simulink model "average_inverter_foc"  (R2023b)
settings: Solver=FixedStepAuto  StartTime=0.0  StopTime=simcfg.stop_time  FixedStep=simcfg.Ts_plant  RelTol=1e-3
InitFcn:
  | motor_control_params
values from neighbouring files (symbols this model uses):
  control = evalin('base', 'control')    [build_vibration_comp_test.m]    (also in evaluate_vibration_comp_test.m; motor_control_params.m = apply_cogging_load_config(control, cogging_load_config); open_cogging_position_scan_model.m = apply_cogging_load_config(control, cfg); open_position_scan_ff_validation_model.m = apply_cogging_load_config(control, cfg))
undefined symbols (not defined in the file or in its folder): inverter, motor, simcfg
libraries: mcbplantlib x1, autolibpmsmexterior x1
settings Model: Creator=user  LastModifiedBy=user

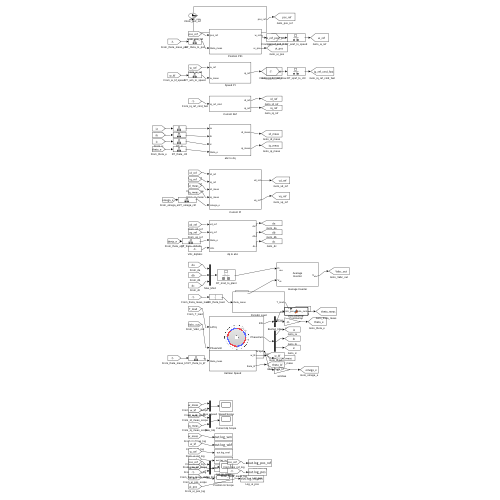
[thumbnail: Simulink's stored preview of the top-level diagram]
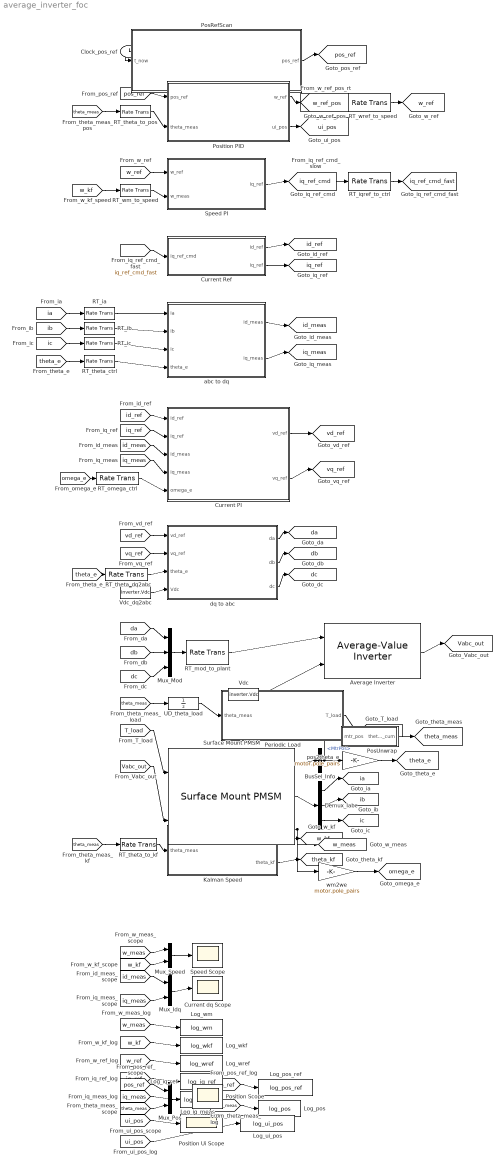
== system average_inverter_foc ==
  Average Inverter : mcbplantlib/Average-Value Inverter
  BusSel_Info : BusSelector  OutputSignals=MtrPos
  Clock_pos_ref : Clock
  Current PI : Subsystem
  Current Ref : Subsystem
  Current dq Scope : Scope
  Demux_Iabc : Demux  Outputs=3
  Kalman Speed : Subsystem
  Log_iq_meas : ToWorkspace  VariableName=log_iq_meas  SaveFormat=Timeseries  SampleTime=-1
  Log_iq_ref : ToWorkspace  VariableName=log_iq_ref  SaveFormat=Timeseries  SampleTime=-1
  Log_pos : ToWorkspace  VariableName=log_pos  SaveFormat=Timeseries  SampleTime=-1
  Log_pos_ref : ToWorkspace  VariableName=log_pos_ref  SaveFormat=Timeseries  SampleTime=-1
  Log_ui_pos : ToWorkspace  VariableName=log_ui_pos  SaveFormat=Timeseries  SampleTime=-1
  Log_wkf : ToWorkspace  VariableName=log_wkf  SaveFormat=Timeseries  SampleTime=-1
  Log_wm : ToWorkspace  VariableName=log_wm  SaveFormat=Timeseries  SampleTime=-1
  Log_wref : ToWorkspace  VariableName=log_wref  SaveFormat=Timeseries  SampleTime=-1
  Mux_Idq : Mux  Inputs=2
  Mux_Mod : Mux  Inputs=3
  Mux_Pos : Mux  Inputs=2
  Mux_Speed : Mux  Inputs=2
  Periodic Load : Subsystem
  PosRefScan : Subsystem
  PosUnwrap : MATLAB Function  TreatAsAtomicUnit=on
  Position PID : Subsystem
  Position Scope : Scope
  Position Ui Scope : Scope
  RT_ia : RateTransition  OutPortSampleTime=simcfg.Ts_ctrl
  RT_ib : RateTransition  OutPortSampleTime=simcfg.Ts_ctrl
  RT_ic : RateTransition  OutPortSampleTime=simcfg.Ts_ctrl
  RT_iqref_to_ctrl : RateTransition  OutPortSampleTime=simcfg.Ts_ctrl
  RT_mod_to_plant : RateTransition  OutPortSampleTime=simcfg.Ts_plant
  RT_omega_ctrl : RateTransition  OutPortSampleTime=simcfg.Ts_ctrl
  RT_theta_ctrl : RateTransition  OutPortSampleTime=simcfg.Ts_ctrl
  RT_theta_dq2abc : RateTransition  OutPortSampleTime=simcfg.Ts_ctrl
  RT_theta_to_kf : RateTransition  OutPortSampleTime=simcfg.Ts_ctrl
  RT_theta_to_pos : RateTransition  OutPortSampleTime=simcfg.Ts_pos
  RT_wm_to_speed : RateTransition  OutPortSampleTime=simcfg.Ts_speed
  RT_wref_to_speed : RateTransition  OutPortSampleTime=simcfg.Ts_speed
  Speed PI : Subsystem
  Speed Scope : Scope
  Surface Mount PMSM : autolibpmsmexterior/Surface Mount PMSM  port_config=Torque  sim_type=Discrete  Ts=simcfg.Ts_plant  P=motor.pole_pairs  Rs=motor.Rs  Ldq_=motor.Ld  KConstText=Permanent flux linkage constant (lambda_pm):  lambda_pm=motor.psi_f  Ke=159.9771  Kt=1.323  mechanical=[motor.J, motor.B, 0]  idq0=[0 0]  theta_init=0  omega_init=0  KConst=motor.psi_f  lambda_pm_calc=motor.psi_f  RefBlkName='autolibpmsmexterior/Surface Mount PMSM'  aMode=5  Ldq="[0.0017      0.0017]"
  UD_theta_load : UnitDelay  SampleTime=simcfg.Ts_plant  HasFrameUpgradeWarning=on
  Vdc : Constant  Value=inverter.Vdc
  Vdc_dq2abc : Constant  Value=inverter.Vdc
  abc to dq : Subsystem
  dq to abc : Subsystem
  pos2theta_e : Gain  Gain=motor.pole_pairs
  wm2we : Gain  Gain=motor.pole_pairs
  tag scope: T_load=global, Vabc_out=global, da=global, db=global, dc=global, ia=global, ib=global, ic=global, id_meas=global, id_ref=global, iq_meas=global, iq_ref=global, iq_ref_cmd=global, iq_ref_cmd_fast=global, omega_e=global, pos_ref=global, theta_e=global, theta_kf=global, theta_meas=global, ui_pos=global, vd_ref=global, vq_ref=global, w_kf=global, w_meas=global, w_ref=global, w_ref_pos=global
  wires:
  Clock_pos_ref/1 -> PosRefScan/1(t_now)
  PosRefScan/1(pos_ref) -> [pos_ref]
  [theta_meas] -> RT_theta_to_pos/1
  [pos_ref] -> Position PID/1(pos_ref)
  RT_theta_to_pos/1 -> Position PID/2(theta_meas)
  Position PID/1(w_ref) -> [w_ref_pos]
  Position PID/2(ui_pos) -> [ui_pos]
  [w_ref_pos] -> RT_wref_to_speed/1
  RT_wref_to_speed/1 -> [w_ref]
  [w_kf] -> RT_wm_to_speed/1
  [w_ref] -> Speed PI/1(w_ref)
  RT_wm_to_speed/1 -> Speed PI/2(w_meas)
  Speed PI/1(iq_ref) -> [iq_ref_cmd]
  [iq_ref_cmd] -> RT_iqref_to_ctrl/1
  RT_iqref_to_ctrl/1 -> [iq_ref_cmd_fast]
  [iq_ref_cmd_fast] -> Current Ref/1(iq_ref_cmd)
  Current Ref/1(id_ref) -> [id_ref]
  Current Ref/2(iq_ref) -> [iq_ref]
  [ia] -> RT_ia/1
  [ib] -> RT_ib/1
  [ic] -> RT_ic/1
  [theta_e] -> RT_theta_ctrl/1
  RT_ia/1 -> abc to dq/1(ia)
  RT_ib/1 -> abc to dq/2(ib)
  RT_ic/1 -> abc to dq/3(ic)
  RT_theta_ctrl/1 -> abc to dq/4(theta_e)
  abc to dq/1(id_meas) -> [id_meas]
  abc to dq/2(iq_meas) -> [iq_meas]
  [omega_e] -> RT_omega_ctrl/1
  [id_ref] -> Current PI/1(id_ref)
  [iq_ref] -> Current PI/2(iq_ref)
  [id_meas] -> Current PI/3(id_meas)
  [iq_meas] -> Current PI/4(iq_meas)
  RT_omega_ctrl/1 -> Current PI/5(omega_e)
  Current PI/1(vd_ref) -> [vd_ref]
  Current PI/2(vq_ref) -> [vq_ref]
  [theta_e] -> RT_theta_dq2abc/1
  [vd_ref] -> dq to abc/1(vd_ref)
  [vq_ref] -> dq to abc/2(vq_ref)
  RT_theta_dq2abc/1 -> dq to abc/3(theta_e)
  Vdc_dq2abc/1 -> dq to abc/4(Vdc)
  dq to abc/1(da) -> [da]
  dq to abc/2(db) -> [db]
  dq to abc/3(dc) -> [dc]
  [da] -> Mux_Mod/1
  [db] -> Mux_Mod/2
  [dc] -> Mux_Mod/3
  Mux_Mod/1 -> RT_mod_to_plant/1
  RT_mod_to_plant/1 -> Average Inverter/1
  Vdc/1 -> Average Inverter/2
  Average Inverter/1 -> [Vabc_out]
  [theta_meas] -> UD_theta_load/1
  UD_theta_load/1 -> Periodic Load/1(theta_meas)
  Periodic Load/1(T_load) -> [T_load]
  [T_load] -> Surface Mount PMSM/1
  [Vabc_out] -> Surface Mount PMSM/2
  Surface Mount PMSM/1 -> BusSel_Info/1
  BusSel_Info/1 -> pos2theta_e/1, PosUnwrap/1(mtr_pos)  "<MtrPos>"
  pos2theta_e/1 -> [theta_e]
  PosUnwrap/1(theta_cum) -> [theta_meas]
  Surface Mount PMSM/2 -> Demux_Iabc/1
  Demux_Iabc/1 -> [ia]
  Demux_Iabc/2 -> [ib]
  Demux_Iabc/3 -> [ic]
  Surface Mount PMSM/3 -> [w_meas], wm2we/1
  wm2we/1 -> [omega_e]
  [theta_meas] -> RT_theta_to_kf/1
  RT_theta_to_kf/1 -> Kalman Speed/1(theta_meas)
  Kalman Speed/1(w_kf) -> [w_kf]
  Kalman Speed/2(theta_kf) -> [theta_kf]
  [w_meas] -> Mux_Speed/1
  [w_kf] -> Mux_Speed/2
  Mux_Speed/1 -> Speed Scope/1
  [id_meas] -> Mux_Idq/1
  [iq_meas] -> Mux_Idq/2
  Mux_Idq/1 -> Current dq Scope/1
  [w_meas] -> Log_wm/1
  [w_kf] -> Log_wkf/1
  [w_ref] -> Log_wref/1
  [iq_ref] -> Log_iq_ref/1
  [iq_meas] -> Log_iq_meas/1
  [ui_pos] -> Position Ui Scope/1
  [ui_pos] -> Log_ui_pos/1
  [pos_ref] -> Mux_Pos/1
  [theta_meas] -> Mux_Pos/2
  Mux_Pos/1 -> Position Scope/1
  [pos_ref] -> Log_pos_ref/1
  [theta_meas] -> Log_pos/1

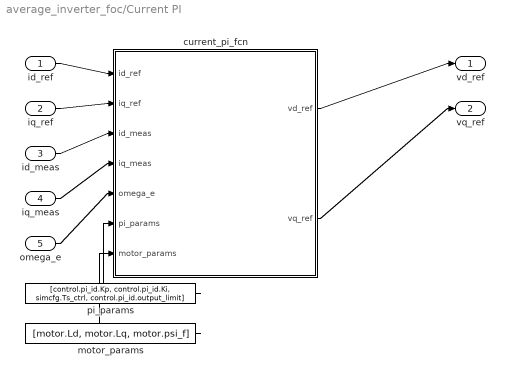
== system average_inverter_foc/Current PI ==
  id_ref : Inport
  iq_ref : Inport  Port=2
  id_meas : Inport  Port=3
  iq_meas : Inport  Port=4
  omega_e : Inport  Port=5
  current_pi_fcn : MATLAB Function  TreatAsAtomicUnit=on
  motor_params : Constant  Value=[motor.Ld, motor.Lq, motor.psi_f]
  pi_params : Constant  Value=[control.pi_id.Kp, control.pi_id.Ki, simcfg.Ts_ctrl, control.pi_id.output_limit]
  vd_ref : Outport
  vq_ref : Outport  Port=2
  wires:
  id_ref/1 -> current_pi_fcn/1(id_ref)
  iq_ref/1 -> current_pi_fcn/2(iq_ref)
  id_meas/1 -> current_pi_fcn/3(id_meas)
  iq_meas/1 -> current_pi_fcn/4(iq_meas)
  omega_e/1 -> current_pi_fcn/5(omega_e)
  pi_params/1 -> current_pi_fcn/6(pi_params)
  motor_params/1 -> current_pi_fcn/7(motor_params)
  current_pi_fcn/1(vd_ref) -> vd_ref/1
  current_pi_fcn/2(vq_ref) -> vq_ref/1

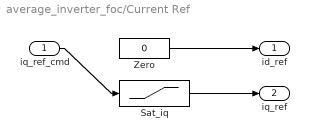
== system average_inverter_foc/Current Ref ==
  iq_ref_cmd : Inport
  Sat_iq : Saturate  UpperLimit=control.iq_ref_limit  LowerLimit=-control.iq_ref_limit
  Zero : Constant  Value=0
  id_ref : Outport
  iq_ref : Outport  Port=2
  wires:
  Zero/1 -> id_ref/1
  iq_ref_cmd/1 -> Sat_iq/1
  Sat_iq/1 -> iq_ref/1

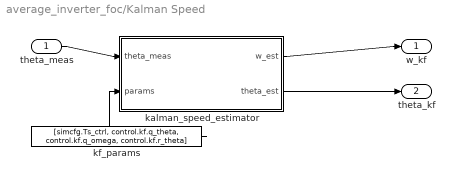
== system average_inverter_foc/Kalman Speed ==
  theta_meas : Inport
  kalman_speed_estimator : MATLAB Function  TreatAsAtomicUnit=on
  kf_params : Constant  Value=[simcfg.Ts_ctrl, control.kf.q_theta, control.kf.q_omega, control.kf.r_theta]
  w_kf : Outport
  theta_kf : Outport  Port=2
  wires:
  theta_meas/1 -> kalman_speed_estimator/1(theta_meas)
  kf_params/1 -> kalman_speed_estimator/2(params)
  kalman_speed_estimator/1(w_est) -> w_kf/1
  kalman_speed_estimator/2(theta_est) -> theta_kf/1

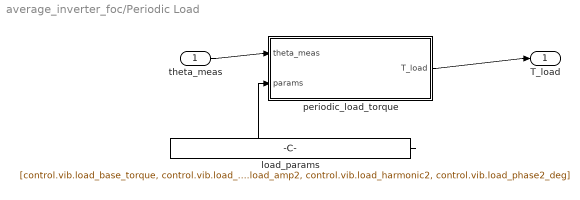
== system average_inverter_foc/Periodic Load ==
  theta_meas : Inport
  load_params : Constant  Value=[control.vib.load_base_torque, control.vib.load_amp1, control.vib.load_harmonic1, control.vib.load_phase1_deg, control.vib.load_amp2, control.vib.load_harmonic2, control.vib.load_phase2_deg]
  periodic_load_torque : MATLAB Function  TreatAsAtomicUnit=on
  T_load : Outport
  wires:
  theta_meas/1 -> periodic_load_torque/1(theta_meas)
  load_params/1 -> periodic_load_torque/2(params)
  periodic_load_torque/1(T_load) -> T_load/1

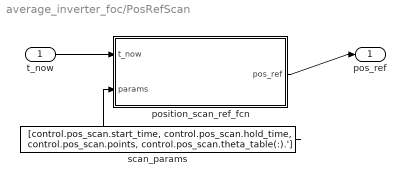
== system average_inverter_foc/PosRefScan ==
  t_now : Inport
  position_scan_ref_fcn : MATLAB Function  TreatAsAtomicUnit=on
  scan_params : Constant  Value=[control.pos_scan.start_time, control.pos_scan.hold_time, control.pos_scan.points, control.pos_scan.theta_table(:).']
  pos_ref : Outport
  wires:
  t_now/1 -> position_scan_ref_fcn/1(t_now)
  scan_params/1 -> position_scan_ref_fcn/2(params)
  position_scan_ref_fcn/1(pos_ref) -> pos_ref/1

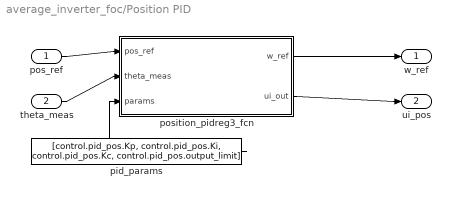
== system average_inverter_foc/Position PID ==
  pos_ref : Inport
  theta_meas : Inport  Port=2
  pid_params : Constant  Value=[control.pid_pos.Kp, control.pid_pos.Ki, control.pid_pos.Kc, control.pid_pos.output_limit]
  position_pidreg3_fcn : MATLAB Function  TreatAsAtomicUnit=on
  w_ref : Outport
  ui_pos : Outport  Port=2
  wires:
  pos_ref/1 -> position_pidreg3_fcn/1(pos_ref)
  theta_meas/1 -> position_pidreg3_fcn/2(theta_meas)
  pid_params/1 -> position_pidreg3_fcn/3(params)
  position_pidreg3_fcn/1(w_ref) -> w_ref/1
  position_pidreg3_fcn/2(ui_out) -> ui_pos/1

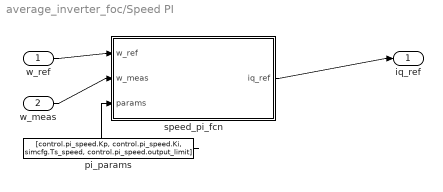
== system average_inverter_foc/Speed PI ==
  w_ref : Inport
  w_meas : Inport  Port=2
  pi_params : Constant  Value=[control.pi_speed.Kp, control.pi_speed.Ki, simcfg.Ts_speed, control.pi_speed.output_limit]
  speed_pi_fcn : MATLAB Function  TreatAsAtomicUnit=on
  iq_ref : Outport
  wires:
  w_ref/1 -> speed_pi_fcn/1(w_ref)
  w_meas/1 -> speed_pi_fcn/2(w_meas)
  pi_params/1 -> speed_pi_fcn/3(params)
  speed_pi_fcn/1(iq_ref) -> iq_ref/1

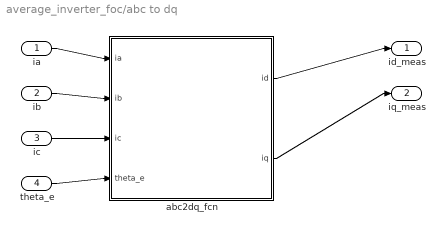
== system average_inverter_foc/abc to dq ==
  ia : Inport
  ib : Inport  Port=2
  ic : Inport  Port=3
  theta_e : Inport  Port=4
  abc2dq_fcn : MATLAB Function  TreatAsAtomicUnit=on
  id_meas : Outport
  iq_meas : Outport  Port=2
  wires:
  ia/1 -> abc2dq_fcn/1(ia)
  ib/1 -> abc2dq_fcn/2(ib)
  ic/1 -> abc2dq_fcn/3(ic)
  theta_e/1 -> abc2dq_fcn/4(theta_e)
  abc2dq_fcn/1(id) -> id_meas/1
  abc2dq_fcn/2(iq) -> iq_meas/1

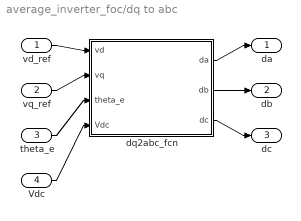
== system average_inverter_foc/dq to abc ==
  vd_ref : Inport
  vq_ref : Inport  Port=2
  theta_e : Inport  Port=3
  Vdc : Inport  Port=4
  dq2abc_fcn : MATLAB Function  TreatAsAtomicUnit=on
  da : Outport
  db : Outport  Port=2
  dc : Outport  Port=3
  wires:
  vd_ref/1 -> dq2abc_fcn/1(vd)
  vq_ref/1 -> dq2abc_fcn/2(vq)
  theta_e/1 -> dq2abc_fcn/3(theta_e)
  Vdc/1 -> dq2abc_fcn/4(Vdc)
  dq2abc_fcn/1(da) -> da/1
  dq2abc_fcn/2(db) -> db/1
  dq2abc_fcn/3(dc) -> dc/1

== matlab function average_inverter_foc/Position PID/position_pidreg3_fcn ==
  data: pos_ref input; w_ref output; theta_meas input; params input; ui_out output
function [w_ref, ui_out] = position_pidreg3_fcn(pos_ref, theta_meas, params)
% Position-loop PIDREG3 controller.
% params = [Kp, Ki_d, Kc, output_limit]

persistent ui out_pre_sat
if isempty(ui)
    ui = 0;
    out_pre_sat = 0;
end

Kp = params(1);
Ki = params(2);
Kc = params(3);
out_lim = params(4);
out_max = out_lim;
out_min = -out_lim;

err = pos_ref - theta_meas;
up = Kp * err;

if Ki == 0
    ui = 0;
    out_pre_sat = up;
    w_ref = min(out_max, max(out_min, out_pre_sat));
    ui_out = 0;
    return;
end

if out_pre_sat > out_max
    if err < 0
        ui = ui + Ki * err;
    else
        ui = ui + Kc * (out_max - out_pre_sat);
    end
elseif out_pre_sat < out_min
    if err > 0
        ui = ui + Ki * err;
    else
        ui = ui + Kc * (out_min - out_pre_sat);
    end
else
    ui = ui + Ki * err;
end

ui = min(out_max, max(out_min, ui));
out_pre_sat = up + ui;
w_ref = min(out_max, max(out_min, out_pre_sat));
ui_out = ui;
end

== matlab function average_inverter_foc/PosRefScan/position_scan_ref_fcn ==
  data: t_now input; pos_ref output; params input
function pos_ref = position_scan_ref_fcn(t_now, params)
% Generate a staircase position reference from a scan table.
% params = [start_time, hold_time, points, theta_table...]

start_time = params(1);
hold_time = max(params(2), eps);
points = max(1, round(params(3)));

table = zeros(points, 1);
available = min(points, numel(params) - 3);
if available > 0
    table(1:available) = params(4:3 + available);
end

if t_now < start_time
    pos_ref = table(1);
    return;
end

idx = 1 + floor((t_now - start_time) / hold_time);
if idx < 1
    idx = 1;
elseif idx > points
    idx = points;
end

pos_ref = table(idx);
end

== matlab function average_inverter_foc/Speed PI/speed_pi_fcn ==
  data: w_ref input; iq_ref output; w_meas input; params input
function iq_ref = speed_pi_fcn(w_ref, w_meas, params)
% Discrete PI speed controller with anti-windup
% params = [Kp, Ki, Ts, output_limit]
persistent int_state
if isempty(int_state)
    int_state = 0;
end
Kp = params(1); Ki = params(2); Ts = params(3); lim = params(4);

err = w_ref - w_meas;
int_state = int_state + Ki * Ts * err;
int_state = max(-lim, min(lim, int_state));
output = Kp * err + int_state;
iq_ref = max(-lim, min(lim, output));

== matlab function average_inverter_foc/abc to dq/abc2dq_fcn ==
  data: ia input; id output; ib input; ic input; theta_e input; iq output
function [id, iq] = abc2dq_fcn(ia, ib, ic, theta_e)
% abc to dq: Clarke + Park transform

% 1. Clarke: abc -> alpha-beta (equal-amplitude)
i_alpha = (2/3) * (ia - 0.5*ib - 0.5*ic);
i_beta  = (2/3) * (sqrt(3)/2*ib - sqrt(3)/2*ic);

% 2. Park: alpha-beta -> dq
id = i_alpha * cos(theta_e) + i_beta * sin(theta_e);
iq = -i_alpha * sin(theta_e) + i_beta * cos(theta_e);

== matlab function average_inverter_foc/Current PI/current_pi_fcn ==
  data: id_ref input; vd_ref output; iq_ref input; id_meas input; iq_meas input; omega_e input; pi_params input; motor_params input; vq_ref output
function [vd_ref, vq_ref] = current_pi_fcn(id_ref, iq_ref, id_meas, iq_meas, omega_e, pi_params, motor_params)
% Discrete PI current controller with cross-coupling decoupling
% pi_params    = [Kp, Ki, Ts, output_limit]
% motor_params = [Ld, Lq, psi_f]
persistent int_d int_q
if isempty(int_d)
    int_d = 0;
    int_q = 0;
end
Kp = pi_params(1); Ki = pi_params(2); Ts = pi_params(3); lim = pi_params(4);
Ld = motor_params(1); Lq = motor_params(2); psi_f = motor_params(3);

% d-axis PI
err_d = id_ref - id_meas;
int_d = int_d + Ki * Ts * err_d;
int_d = max(-lim, min(lim, int_d));
vd_pi = Kp * err_d + int_d;

% q-axis PI
err_q = iq_ref - iq_meas;
int_q = int_q + Ki * Ts * err_q;
int_q = max(-lim, min(lim, int_q));
vq_pi = Kp * err_q + int_q;

% Cross-coupling decoupling
vd_dec = -omega_e * Lq * iq_meas;
vq_dec = omega_e * (Ld * id_meas + psi_f);

% Output
vd_ref = vd_pi + vd_dec;
vq_ref = vq_pi + vq_dec;

== matlab function average_inverter_foc/dq to abc/dq2abc_fcn ==
  data: vd input; da output; vq input; theta_e input; Vdc input; db output; dc output
function [da, db, dc] = dq2abc_fcn(vd, vq, theta_e, Vdc)
% dq -> 占空比: 逆Park + 逆Clarke + SVPWM + 归一化

% 1. 逆Park: dq -> alpha-beta
v_alpha = vd * cos(theta_e) - vq * sin(theta_e);
v_beta  = vd * sin(theta_e) + vq * cos(theta_e);

% 2. 逆Clarke: alpha-beta -> abc
va = v_alpha;
vb = -0.5 * v_alpha + sqrt(3)/2 * v_beta;
vc = -0.5 * v_alpha - sqrt(3)/2 * v_beta;

% 3. SVPWM零序注入
v_max = max(max(va, vb), vc);
v_min = min(min(va, vb), vc);
v_n0  = -0.5 * (v_max + v_min);
va = va + v_n0;
vb = vb + v_n0;
vc = vc + v_n0;

%% 4. 占空比 [0,1]
da = va / Vdc + 0.5;
db = vb / Vdc + 0.5;
dc = vc / Vdc + 0.5;

== matlab function average_inverter_foc/Periodic Load/periodic_load_torque ==
  data: theta_meas input; T_load output; params input
function T_load = periodic_load_torque(theta_meas, params)
% Synthetic compressor-like periodic load torque profile.
%
% params = [base, amp1, harmonic1, phase1_deg, amp2, harmonic2, phase2_deg]

base = params(1);
amp1 = params(2);
harmonic1 = params(3);
phase1 = params(4) * pi / 180;
amp2 = params(5);
harmonic2 = params(6);
phase2 = params(7) * pi / 180;

theta_wrap = mod(theta_meas, 2 * pi);
if theta_wrap < 0
    theta_wrap = theta_wrap + 2 * pi;
end

T_load = base + ...
    amp1 * sin(harmonic1 * theta_wrap + phase1) + ...
    amp2 * sin(harmonic2 * theta_wrap + phase2);
end

== matlab function average_inverter_foc/PosUnwrap ==
  data: mtr_pos input; theta_cum output
function theta_cum = pos_unwrap(mtr_pos)
% Unwrap MtrPos [0,2pi) to cumulative angle
persistent prev_pos revs
if isempty(prev_pos)
    prev_pos = mtr_pos;
    revs = 0;
end
delta = mtr_pos - prev_pos;
if delta < -pi        % 正转过零: 0->2pi 跳到 2pi->0
    revs = revs + 1;
elseif delta > pi     % 反转过零
    revs = revs - 1;
end
prev_pos = mtr_pos;
theta_cum = mtr_pos + revs * 2 * pi;

== matlab function average_inverter_foc/Kalman Speed/kalman_speed_estimator ==
  data: theta_meas input; w_est output; params input; theta_est output
function [w_est, theta_est] = kalman_speed_estimator(theta_meas, params)
% Discrete Kalman filter for speed estimation from position measurement.
%
% State:       x = [theta; omega]
% Model:       x(k+1) = A * x(k),  A = [1 Ts; 0 1]
% Measurement: z = H * x,           H = [1 0]
%
% params = [Ts, q_theta, q_omega, r_theta]
%   Ts      — sample time
%   q_theta — process noise on position (tune small, e.g. 1e-6)
%   q_omega — process noise on speed    (tune larger, e.g. 0.1)
%   r_theta — measurement noise on position (e.g. 1e-4)

persistent x_est P
if isempty(x_est)
    x_est = [0; 0];
    P = eye(2);
end

Ts = params(1);
Q  = [params(2) 0; 0 params(3)];
R  = params(4);

A = [1 Ts; 0 1];
H = [1 0];

% --- Predict ---
x_pred = A * x_est;
P_pred = A * P * A' + Q;

% --- Update ---
S = H * P_pred * H' + R;
K = P_pred * H' / S;
y_innov = theta_meas - H * x_pred;
x_est = x_pred + K * y_innov;
P = (eye(2) - K * H) * P_pred;

% --- Output ---
theta_est = x_est(1);
w_est     = x_est(2);
